simulink model "robotPrototype"  (R2021a)
settings: Solver=ode15s  StartTime=0.0  StopTime=simTime
model workspace: external: MAT-File (data not in the file)
values from neighbouring files (symbols this model uses):
  controlLim = [0.15 3 3]    [simulinkModelParam.mat]
  controlWeight = [0.75 0.6 0.5]    [simulinkModelParam.mat]
  delta = 0.3    [robotParameters.m]    (also in simulinkModelParam.mat = 0.25)
  deltaPlus = 0.20    (= 0.2)    [robotParameters.m]    (also in simulinkModelParam.mat = 0.15)
  den_CoP = [1 -1.84477840502 0.855986791935]    [simulinkModelParam.mat]
  den_zddot = [1 -1.92894226325 0.931381682127]    [simulinkModelParam.mat]
  f_0 = [1,1; deltaPlus-CoM_0(1), -(delta-deltaPlus+CoM_0(1))]\[m*9.81/2;0]    [robotParameters.m]
  f_sample = 500    [robotParameters.m]    (also in simulinkModelParam.mat = 1000)
  filterCoef = 50    [robotParameters.m]    (also in simulinkModelParam.mat = 1000)
  foot_x = delta    (= 0.3)    [robotParameters.m]    (also in simulinkModelParam.mat = 0.25)
  foot_y = delta/3    (= 0.1)    [robotParameters.m]    (also in simulinkModelParam.mat = 0.0833333333333)
  foot_z = 0.03    [robotParameters.m]    (also in simulinkModelParam.mat = 0.02)
  kd_ank = 0    [robotParameters.m]    (also in simulinkModelParam.mat)
  kd_hip = 250    [robotParameters.m]    (also in simulinkModelParam.mat = 12)
  kd_knee1 = 0.02    [robotParameters.m]    (also in simulinkModelParam.mat = 0)
  kd_knee2 = 500    [robotParameters.m]    (also in simulinkModelParam.mat = 150)
  ki_ank = 1800    [robotParameters.m]    (also in simulinkModelParam.mat = 500)
  ki_hip = 0    [robotParameters.m]    (also in simulinkModelParam.mat)
  ki_knee1 = 0    [robotParameters.m]    (also in simulinkModelParam.mat = 0.5)
  ki_knee2 = 0    [robotParameters.m]    (also in simulinkModelParam.mat)
  kp_ank = 375    [robotParameters.m]    (also in simulinkModelParam.mat = 325)
  kp_hip = 500    [robotParameters.m]    (also in simulinkModelParam.mat = 25)
  kp_knee1 = 8    [robotParameters.m]    (also in simulinkModelParam.mat = 3)
  kp_knee2 = 1000    [robotParameters.m]    (also in simulinkModelParam.mat = 300)
  L = 0.94*2*legLength    (= 0.7896)    [robotParameters.m]    (also in simulinkModelParam.mat = 0.72)
  legLength = param(1)    [forwardKin.m]    (also in robotParameters.m = 0.42; simulinkModelParam.mat = 0.4)
  legWidth = 0.08    [robotParameters.m]    (also in simulinkModelParam.mat = 0.05)
  limbThickness = 0.05    [robotParameters.m]    (also in simulinkModelParam.mat = 0.025)
  m = param(3)    [forwardKin.m]    (also in robotParameters.m = 70; simulinkModelParam.mat = 25)
  modelProperties = [25 0.5781 0.72]    [simulinkModelParam.mat]
  N = length(theta)    [robotParameters.m]
  num_CoP = [0.00280209672777 0.00560419345555 0.00280209672777]    [simulinkModelParam.mat]
  num_zddot = [0.000609854718717 0.00121970943743 0.000609854718717]    [simulinkModelParam.mat]
  p = 28    [simulinkModelParam.mat]
  pushDur = 0.1    [compareReducedOrderModels.m]    (also in simulinkModelParam.mat; startUpBalanceRobot.m)
  pushForce = pushForce - 2*pushStep    (= 0)    [compareReducedOrderModels.m]    (also in startUpBalanceRobot.m = 494)
  pushOnset = 0.2    [compareReducedOrderModels.m]    (also in simulinkModelParam.mat; startUpBalanceRobot.m)
  segmentMass = struct('torso',0.681, 'thigh', 0.2, 'shank', 0.09, 'foot', 0.029)    [robotParameters.m]
  stateLim = [0.15 1.57079632679 0.8 0.55 1.622 0.3]    [simulinkModelParam.mat]
  stateWeight = [3 0.5 0.3 9 0.25 0.09]    [simulinkModelParam.mat]
  support_x = 2.5    [robotParameters.m]    (also in simulinkModelParam.mat)
  support_y = 2.5    [robotParameters.m]    (also in simulinkModelParam.mat)
  support_z = 0.1    [robotParameters.m]    (also in simulinkModelParam.mat)
  torsoCoM = param(2)    [forwardKin.m]    (also in robotParameters.m = 0.235; simulinkModelParam.mat = 0.1875)
  torsoLength = 0.47    [robotParameters.m]    (also in simulinkModelParam.mat = 0.25)
  zmax = (2*legLength)*sin(acos(0.2/(2*legLength)))+ankleOffset    [robotParameters.m]    (also in simulinkModelParam.mat = 0.8)
  zmin = 0.6+ ankleOffset    (= 0.67)    [robotParameters.m]    (also in simulinkModelParam.mat = 0.6)
undefined symbols (not defined in the file or in its folder): controlRateWeight, den_qdot, nlobjLIP, num_qdot, X, Y, Z
libraries: sm_lib x27, nesl_utility x19, pid_lib x16, robotmaniplib x16, simulink_extras x16, mpclib x4, Contact_Forces_Lib x4, simulink x2
(part 2 of 3)

== system robotPrototype/Robot/Torso ==
  CoM to Hip : sm_lib/Frames and Transforms/Rigid Transform  TranslationMethod=StandardAxis  TranslationStandardOffset=torsoLength-torsoCoM  TranslationLengthUnit=m  TranslationStandardAxis=-Z  TranslationCartesianOffset=[0 0 0]  TranslationROffset=0  TranslationROffsetUnits=m  TranslationZOffset=0  TranslationZOffsetUnits=m  TranslationThetaOffset=0  TranslationThetaOffsetUnits=deg  RotationMethod=StandardAxis  RotationAngleUnits=deg  RotationStandardAxis=+X  RotationAngle=0  RotationArbitraryAxis=[0 0 1]  FollAlignAxisA=+X  BaseAlignAxisA=+Y  FollAlignAxisB=+Y  BaseAlignAxisB=+Z  RotationSequenceAxes=FollowerAxes  RotationSequence=XYX  RotationSequenceAngles=[0 0 0]  RotationSequenceAnglesUnits=deg  RotationMatrix=[1 0 0; 0 1 0; 0 0 1]
  CoM torso : sm_lib/Frames and Transforms/Rigid Transform  TranslationMethod=StandardAxis  TranslationStandardOffset=torsoCoM  TranslationLengthUnit=m  TranslationStandardAxis=-Y  TranslationCartesianOffset=[0 0 0]  TranslationROffset=0  TranslationROffsetUnits=m  TranslationZOffset=0  TranslationZOffsetUnits=m  TranslationThetaOffset=0  TranslationThetaOffsetUnits=deg  RotationMethod=StandardAxis  RotationAngleUnits=deg  RotationStandardAxis=+X  RotationAngle=-90  RotationArbitraryAxis=[0 0 1]  FollAlignAxisA=+X  BaseAlignAxisA=+Y  FollAlignAxisB=+Y  BaseAlignAxisB=+Z  RotationSequenceAxes=FollowerAxes  RotationSequence=XYX  RotationSequenceAngles=[0 0 0]  RotationSequenceAnglesUnits=deg  RotationMatrix=[1 0 0; 0 1 0; 0 0 1]
  Hip to joint orientation : sm_lib/Frames and Transforms/Rigid Transform  TranslationMethod=None  TranslationStandardOffset=0  TranslationLengthUnit=m  TranslationStandardAxis=+Z  TranslationCartesianOffset=[0 0 0]  TranslationROffset=0  TranslationROffsetUnits=m  TranslationZOffset=0  TranslationZOffsetUnits=m  TranslationThetaOffset=0  TranslationThetaOffsetUnits=deg  RotationMethod=StandardAxis  RotationAngleUnits=deg  RotationStandardAxis=+X  RotationAngle=90  RotationArbitraryAxis=[0 0 1]  FollAlignAxisA=+X  BaseAlignAxisA=+Y  FollAlignAxisB=+Y  BaseAlignAxisB=+Z  RotationSequenceAxes=FollowerAxes  RotationSequence=XYX  RotationSequenceAngles=[0 0 0]  RotationSequenceAnglesUnits=deg  RotationMatrix=[1 0 0; 0 1 0; 0 0 1]
  Planar Joint to Torso : sm_lib/Frames and Transforms/Rigid Transform  TranslationMethod=None  TranslationStandardOffset=0  TranslationLengthUnit=m  TranslationStandardAxis=+Z  TranslationCartesianOffset=[0 0 0]  TranslationROffset=0  TranslationROffsetUnits=m  TranslationZOffset=0  TranslationZOffsetUnits=m  TranslationThetaOffset=0  TranslationThetaOffsetUnits=deg  RotationMethod=None  RotationAngleUnits=deg  RotationStandardAxis=+Z  RotationAngle=0.0  RotationArbitraryAxis=[0 0 1]  FollAlignAxisA=+X  BaseAlignAxisA=+Y  FollAlignAxisB=+Y  BaseAlignAxisB=+Z  RotationSequenceAxes=FollowerAxes  RotationSequence=XYX  RotationSequenceAngles=[0 0 0]  RotationSequenceAnglesUnits=deg  RotationMatrix=[1 0 0; 0 1 0; 0 0 1]
  Torso : sm_lib/Body Elements/Extruded Solid  GraphicAmbientColor=[0.15 0.15 0.15 1.0]  BasedOnType=Mass  CenterOfMass=[0 -torsoCoM 0]  CenterOfMassUnits=m  GraphicDiffuseColor=[0.0 0.0 1.0]  ExportConvexHullGeometry=off  ExtrusionCrossSection=torso_xy  ExtrusionCrossSectionUnits=m  Density=1000  DensityUnits=kg/m^3  DoExposeReferenceFrame=on  GraphicEmissiveColor=[0.0 0.0 0.0 1.0]  ExportEntireGeometry=off  ExtrusionLength=limbThickness+0.02  ExtrusionLengthUnits=m  ExtrusionType=General  SerializedFrames=<Frames/>  MarkerShape=Sphere  MarkerSize=10  GraphicType=FromGeometry  InertiaType=Custom  Mass=segmentMass.torso*m  MassUnits=kg  MomentsOfInertia=[1.367 0.094 (8 - segmentMass.torso*m*(torsoCoM)^2 )]  MomentsOfInertiaUnits=kg*m^2  PolygonNumSides=3  GraphicOpacity=1.0  PolygonOuterRadius=1  PolygonOuterRadiusUnits=m  ProductsOfInertia=[0 0 0]  ProductsOfInertiaUnits=kg*m^2  GraphicShininess=75  GraphicSpecularColor=[0.5 0.5 0.5 1.0]  GraphicVisPropType=SimpleVisualProperties
  Hip Frame : PMIOPort  Side=Left
  Planar Joint : PMIOPort  Port=2  Side=Left
  Hip Joint : PMIOPort  Port=3  Side=Right
  Disturbance : PMIOPort  Port=4  Side=Left
  connections:
  Torso/RConn1 -- Planar Joint to Torso/RConn1 -- CoM torso/LConn1
  Hip Frame/RConn1 -- Disturbance/RConn1 -- Hip to joint orientation/LConn1 -- CoM to Hip/RConn1
  Planar Joint to Torso/LConn1 -- Planar Joint/RConn1
  CoM to Hip/LConn1 -- CoM torso/RConn1
  Hip Joint/RConn1 -- Hip to joint orientation/RConn1

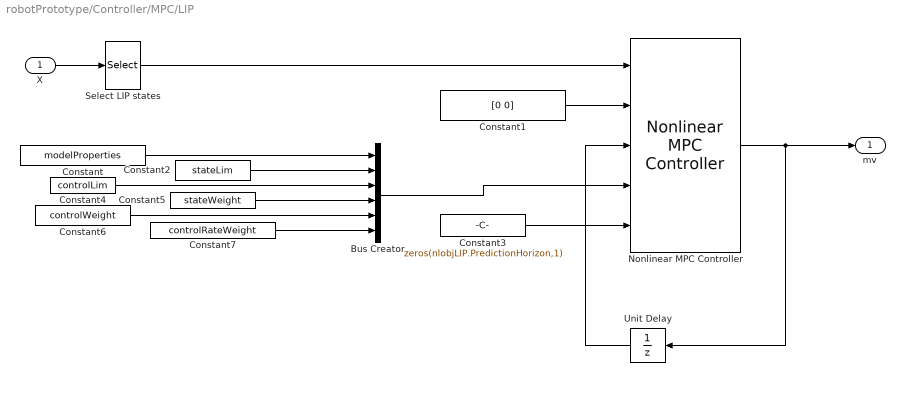
== system robotPrototype/Controller/MPC/LIP ==
  X : Inport
  Bus Creator : BusCreator  Inputs=6  OutDataTypeStr=Bus: myBusObjectLIP  NonVirtualBus=on
      settings: InheritFromInputs=off
  Constant : Constant  Value=modelProperties
  Constant1 : Constant  Value=[0 0]  VectorParams1D=off  OutDataTypeStr=double
  Constant2 : Constant  Value=stateLim
  Constant3 : Constant  Value=zeros(nlobjLIP.PredictionHorizon,1)
  Constant4 : Constant  Value=controlLim
  Constant5 : Constant  Value=stateWeight
  Constant6 : Constant  Value=controlWeight
  Constant7 : Constant  Value=controlRateWeight
  Nonlinear MPC Controller : mpclib/Nonlinear MPC Controller  SCDEnableBlockLinearizationSpecification=on  nlmpcobj=nlobjLIP  UseObjectTs=on  UseMEX=off  md_enabled=off  mvtarget_enabled=on  param_enabled=on  cost_enabled=off  mvseq_enabled=off  stateseq_enabled=off  ovseq_enabled=off  slack_enabled=off  status_enabled=off  ov_min=off  ov_max=off  mv_min=off  mv_max=off  mvrate_min=off  mvrate_max=off  state_min=off  state_max=off  ov_weight=off  mv_weight=off  mvrate_weight=off  ecr_weight=off  nlp_initialize=off
  Select LIP states : Selector  InputPortWidth=6  IndexOptions=Index vector (dialog)  Indices=[1 4]  OutputSizes=1
  Unit Delay : UnitDelay  SampleTime=-1  HasFrameUpgradeWarning=on
  mv : Outport
  wires:
  Bus Creator/1 -> Nonlinear MPC Controller/4
  Constant3/1 -> Nonlinear MPC Controller/5
  Unit Delay/1 -> Nonlinear MPC Controller/3
  Constant1/1 -> Nonlinear MPC Controller/2
  Nonlinear MPC Controller/1 -> Unit Delay/1, mv/1
  X/1 -> Select LIP states/1
  Select LIP states/1 -> Nonlinear MPC Controller/1
  Constant5/1 -> Bus Creator/4
  Constant4/1 -> Bus Creator/3
  Constant2/1 -> Bus Creator/2
  Constant/1 -> Bus Creator/1
  Constant6/1 -> Bus Creator/5
  Constant7/1 -> Bus Creator/6

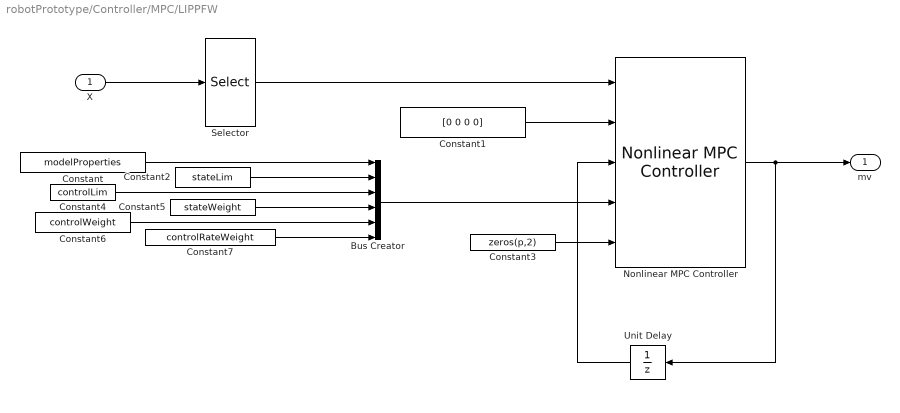
== system robotPrototype/Controller/MPC/LIPPFW ==
  X : Inport
  Bus Creator : BusCreator  Inputs=6  OutDataTypeStr=Bus: myBusObjectLIPPFW  NonVirtualBus=on
      settings: InheritFromInputs=off
  Constant : Constant  Value=modelProperties
  Constant1 : Constant  Value=[0 0 0 0]  VectorParams1D=off  OutDataTypeStr=double
  Constant2 : Constant  Value=stateLim
  Constant3 : Constant  Value=zeros(p,2)
  Constant4 : Constant  Value=controlLim
  Constant5 : Constant  Value=stateWeight
  Constant6 : Constant  Value=controlWeight
  Constant7 : Constant  Value=controlRateWeight
  Nonlinear MPC Controller : mpclib/Nonlinear MPC Controller  SCDEnableBlockLinearizationSpecification=on  nlmpcobj=nlobjLIPPFW  UseObjectTs=on  UseMEX=off  md_enabled=off  mvtarget_enabled=on  param_enabled=on  cost_enabled=off  mvseq_enabled=off  stateseq_enabled=off  ovseq_enabled=off  slack_enabled=off  status_enabled=off  ov_min=off  ov_max=off  mv_min=off  mv_max=off  mvrate_min=off  mvrate_max=off  state_min=off  state_max=off  ov_weight=off  mv_weight=off  mvrate_weight=off  ecr_weight=off  nlp_initialize=off
  Selector : Selector  InputPortWidth=6  IndexOptions=Index vector (dialog)  Indices=[1 2 4 5]  OutputSizes=1
  Unit Delay : UnitDelay  SampleTime=-1  HasFrameUpgradeWarning=on
  mv : Outport
  wires:
  Unit Delay/1 -> Nonlinear MPC Controller/3
  Constant1/1 -> Nonlinear MPC Controller/2
  Nonlinear MPC Controller/1 -> mv/1, Unit Delay/1
  Bus Creator/1 -> Nonlinear MPC Controller/4
  Constant3/1 -> Nonlinear MPC Controller/5
  Constant5/1 -> Bus Creator/4
  Constant4/1 -> Bus Creator/3
  Constant2/1 -> Bus Creator/2
  Constant/1 -> Bus Creator/1
  Constant6/1 -> Bus Creator/5
  X/1 -> Selector/1
  Selector/1 -> Nonlinear MPC Controller/1
  Constant7/1 -> Bus Creator/6

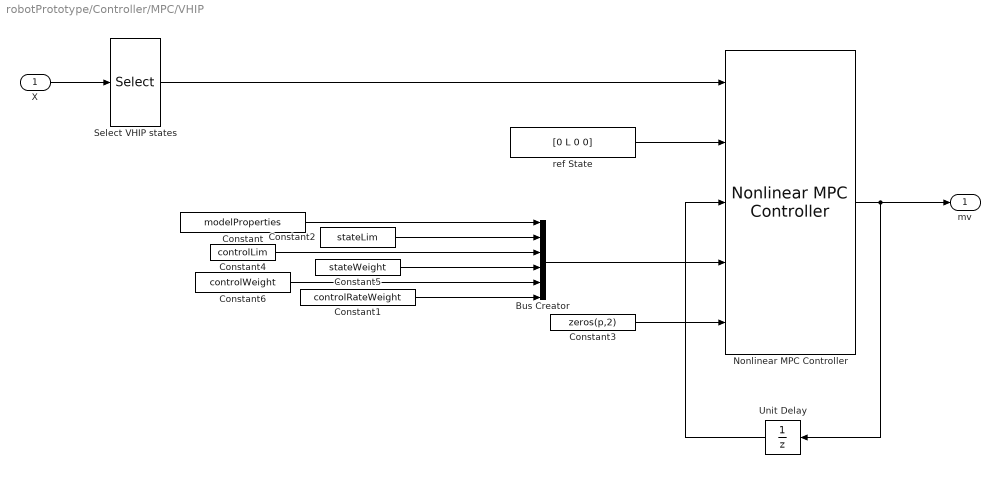
== system robotPrototype/Controller/MPC/VHIP ==
  X : Inport
  Bus Creator : BusCreator  Inputs=6  OutDataTypeStr=Bus: myBusObjectVHIP  NonVirtualBus=on
      settings: InheritFromInputs=off
  Constant : Constant  Value=modelProperties
  Constant1 : Constant  Value=controlRateWeight
  Constant2 : Constant  Value=stateLim
  Constant3 : Constant  Value=zeros(p,2)
  Constant4 : Constant  Value=controlLim
  Constant5 : Constant  Value=stateWeight
  Constant6 : Constant  Value=controlWeight
  Nonlinear MPC Controller : mpclib/Nonlinear MPC Controller  SCDEnableBlockLinearizationSpecification=on  nlmpcobj=nlobjVHIP  UseObjectTs=on  UseMEX=off  md_enabled=off  mvtarget_enabled=on  param_enabled=on  cost_enabled=off  mvseq_enabled=off  stateseq_enabled=off  ovseq_enabled=off  slack_enabled=off  status_enabled=off  ov_min=off  ov_max=off  mv_min=off  mv_max=off  mvrate_min=off  mvrate_max=off  state_min=off  state_max=off  ov_weight=off  mv_weight=off  mvrate_weight=off  ecr_weight=off  nlp_initialize=off
  Select VHIP states : Selector  InputPortWidth=6  IndexOptions=Index vector (dialog)  Indices=[1 3 4 6]  OutputSizes=1
  Unit Delay : UnitDelay  SampleTime=-1  HasFrameUpgradeWarning=on
  ref State : Constant  Value=[0 L 0 0]  VectorParams1D=off  OutDataTypeStr=double
  mv : Outport
  wires:
  Unit Delay/1 -> Nonlinear MPC Controller/3
  ref State/1 -> Nonlinear MPC Controller/2
  Nonlinear MPC Controller/1 -> Unit Delay/1, mv/1
  Bus Creator/1 -> Nonlinear MPC Controller/4
  Constant3/1 -> Nonlinear MPC Controller/5
  X/1 -> Select VHIP states/1
  Select VHIP states/1 -> Nonlinear MPC Controller/1
  Constant5/1 -> Bus Creator/4
  Constant/1 -> Bus Creator/1
  Constant4/1 -> Bus Creator/3
  Constant2/1 -> Bus Creator/2
  Constant6/1 -> Bus Creator/5
  Constant1/1 -> Bus Creator/6

== system robotPrototype/Controller/MPC/VHIPPFW ==
  X : Inport
  Bus Creator : BusCreator  Inputs=6  OutDataTypeStr=Bus: myBusObjectVHIPPFW  NonVirtualBus=on
      settings: InheritFromInputs=off
  Constant : Constant  Value=modelProperties
  Constant1 : Constant  Value=controlRateWeight
  Constant2 : Constant  Value=stateLim
  Constant3 : Constant  Value=zeros(p,3)
  Constant4 : Constant  Value=controlLim
  Constant5 : Constant  Value=stateWeight
  Constant6 : Constant  Value=controlWeight
  Nonlinear MPC Controller : mpclib/Nonlinear MPC Controller  SCDEnableBlockLinearizationSpecification=on  nlmpcobj=nlobjVHIPPFW  UseObjectTs=on  UseMEX=off  md_enabled=off  mvtarget_enabled=on  param_enabled=on  cost_enabled=off  mvseq_enabled=off  stateseq_enabled=off  ovseq_enabled=off  slack_enabled=off  status_enabled=off  ov_min=off  ov_max=off  mv_min=off  mv_max=off  mvrate_min=off  mvrate_max=off  state_min=off  state_max=off  ov_weight=off  mv_weight=off  mvrate_weight=off  ecr_weight=off  nlp_initialize=off
  Unit Delay : UnitDelay  SampleTime=-1  HasFrameUpgradeWarning=on
  refState : Constant  Value=[0 0 L 0 0 0]  VectorParams1D=off  OutDataTypeStr=double
  mv : Outport
  wires:
  Bus Creator/1 -> Nonlinear MPC Controller/4
  Constant3/1 -> Nonlinear MPC Controller/5
  Constant2/1 -> Bus Creator/2
  Constant/1 -> Bus Creator/1
  X/1 -> Nonlinear MPC Controller/1
  Unit Delay/1 -> Nonlinear MPC Controller/3
  refState/1 -> Nonlinear MPC Controller/2
  Nonlinear MPC Controller/1 -> mv/1, Unit Delay/1
  Constant4/1 -> Bus Creator/3
  Constant5/1 -> Bus Creator/4
  Constant6/1 -> Bus Creator/5
  Constant1/1 -> Bus Creator/6

== system robotPrototype/Controller/Variant Subsystem/LIP ==
  mv : Inport
  measureData : Inport  Port=2
  Bus Creator : BusCreator  Inputs=3
  Bus Selector : BusSelector  OutputSignals=CoP,jointPos,state,ContactForces,jointAng
  Demux2 : Demux  Outputs=3
  Feedback Correction : Subsystem
  Inverse Dynamics1 : Subsystem
  jointTorque : Outport
  wires:
  measureData/1 -> Bus Selector/1
  Demux2/1 -> Bus Creator/1  "ankle"
  Demux2/2 -> Bus Creator/2  "knee"
  Demux2/3 -> Bus Creator/3  "hip"
  Bus Creator/1 -> jointTorque/1
  mv/1 -> Feedback Correction/1(mpc controls)
  Bus Selector/1 -> Feedback Correction/2(<CoP>)  "<CoP>"
  Bus Selector/2 -> Feedback Correction/3(<jointPos>)  "<jointPos>"
  Bus Selector/3 -> Feedback Correction/4(<state>)  "<state>"
  Feedback Correction/1(tau correction) -> Inverse Dynamics1/1(tau corrective)
  Inverse Dynamics1/1(tau compesation) -> Demux2/1
  Bus Selector/5 -> Inverse Dynamics1/2(<jointAng>)  "<jointAng>"
  Bus Selector/4 -> Feedback Correction/5(footContact)  "<ContactForces>"

== system robotPrototype/Controller/Variant Subsystem/LIPPFW ==
  mv : Inport
  measureData : Inport  Port=2
  Bus Creator : BusCreator  Inputs=3
  Bus Selector : BusSelector  OutputSignals=CoP,jointPos,jointAng,ContactForces
  Demux : Demux  Outputs=3
  Feedback Compensation : Subsystem
  Inverse Dynamics : Subsystem
  jointTorque : Outport
  wires:
  measureData/1 -> Bus Selector/1
  Bus Creator/1 -> jointTorque/1
  Demux/3 -> Bus Creator/3  "hip"
  mv/1 -> Feedback Compensation/1(mpc control)
  Bus Selector/1 -> Feedback Compensation/2(<CoP>)  "<CoP>"
  Bus Selector/2 -> Feedback Compensation/3(<jointPos>)  "<jointPos>"
  Demux/1 -> Bus Creator/1  "ankle"
  Demux/2 -> Bus Creator/2  "knee"
  Feedback Compensation/1(tau corrective) -> Inverse Dynamics/1(tau corrective)
  Inverse Dynamics/1(tau compesation) -> Demux/1
  Bus Selector/3 -> Inverse Dynamics/2(<jointAng>)  "<jointAng>"
  Bus Selector/4 -> Feedback Compensation/4(Heal Normal Force)  "<ContactForces>"

== system robotPrototype/Controller/Variant Subsystem/VHIP ==
  mv : Inport
  measureData : Inport  Port=2
  Bus Creator : BusCreator  Inputs=3
  Bus Selector : BusSelector  OutputSignals=state,CoP,zddot,ContactForces,jointAng
  Demux2 : Demux  Outputs=3
  Feedback Correction : Subsystem
  Inverse Dynamics : Subsystem
  jointTorque : Outport
  wires:
  measureData/1 -> Bus Selector/1
  Bus Creator/1 -> jointTorque/1
  Demux2/1 -> Bus Creator/1  "ankle"
  Demux2/2 -> Bus Creator/2  "knee"
  Demux2/3 -> Bus Creator/3  "hip"
  mv/1 -> Feedback Correction/1(mpc controls)
  Bus Selector/1 -> Feedback Correction/2(<state>)  "<state>"
  Bus Selector/2 -> Feedback Correction/3(<CoP>)  "<CoP>"
  Bus Selector/3 -> Feedback Correction/4(<zddot>)  "<zddot>"
  Bus Selector/5 -> Inverse Dynamics/2(<jointAng>)  "<jointAng>"
  Inverse Dynamics/1(tau compesation) -> Demux2/1
  Feedback Correction/1(Tau correction) -> Inverse Dynamics/1(tau corrective)
  Bus Selector/4 -> Feedback Correction/5(footContact)  "<ContactForces>"

== system robotPrototype/Controller/Variant Subsystem/VIPPFW ==
  mv : Inport
  measureData : Inport  Port=2
  Bus Creator : BusCreator  Inputs=3
  Bus Selector : BusSelector  OutputSignals=CoP,zddot,jointPos,ContactForces,jointAng
  Bus Selector1 : BusSelector  OutputSignals=X_hip
  Demux : Demux  Outputs=3
  Demux1 : Demux  Outputs=2
  Inverse Dynamics : Subsystem
  Terminator : Terminator
  feedback correction : Subsystem
  jointTorque : Outport
  wires:
  Bus Creator/1 -> jointTorque/1
  measureData/1 -> Bus Selector/1
  Bus Selector/5 -> Inverse Dynamics/2(<jointAng>)  "<jointAng>"
  mv/1 -> feedback correction/1(mpc controls)
  Bus Selector/1 -> feedback correction/2(<CoP>)  "<CoP>"
  Bus Selector/2 -> feedback correction/3(<zddot>)  "<zddot>"
  Demux/1 -> Bus Creator/1  "ankle"
  Demux/2 -> Bus Creator/2  "knee"
  Demux/3 -> Bus Creator/3  "hip"
  Bus Selector/3 -> Bus Selector1/1  "<jointPos>"
  Bus Selector1/1 -> Demux1/1  "<X_hip>"
  Demux1/1 -> Terminator/1
  Demux1/2 -> feedback correction/4(z)
  Inverse Dynamics/1(tau compesation) -> Demux/1
  feedback correction/1(tau correction) -> Inverse Dynamics/1(tau corrective)
  Bus Selector/4 -> feedback correction/5(footContact)  "<ContactForces>"

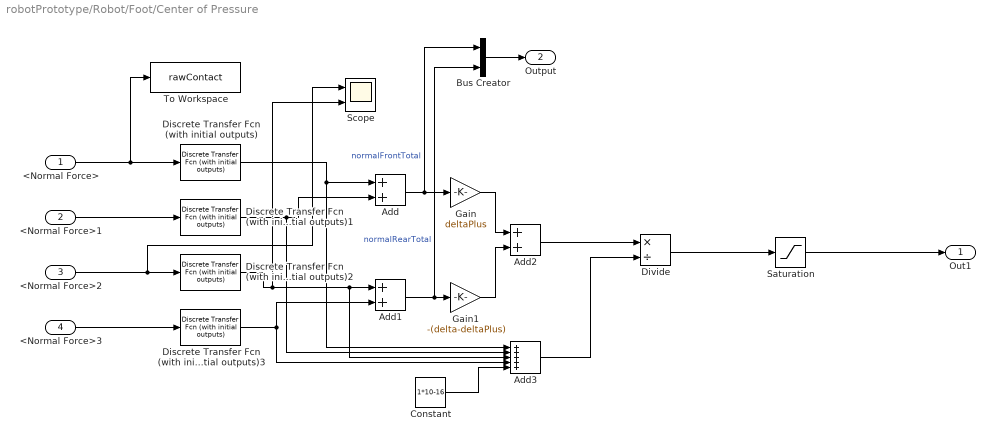
== system robotPrototype/Robot/Foot/Center of Pressure ==
  <Normal Force> : Inport
  <Normal Force>1 : Inport  Port=2
  <Normal Force>2 : Inport  Port=3
  <Normal Force>3 : Inport  Port=4
  Add : Sum
  Add1 : Sum
  Add2 : Sum
  Add3 : Sum  Inputs=+++++
  Bus Creator : BusCreator  Inputs=2
  Constant : Constant  Value=1*10-16
  Discrete Transfer Fcn (with initial outputs) : simulink_extras/Additional Discrete/Discrete Transfer Fcn (with initial outputs)  N=num_CoP  D=den_CoP  U0=0  Y0=f_0(1)  TS=1/f_sample
      settings: SourceProductBaseCode=SL
  Discrete Transfer Fcn (with initial outputs)1 : simulink_extras/Additional Discrete/Discrete Transfer Fcn (with initial outputs)  N=num_CoP  D=den_CoP  U0=0  Y0=f_0(1)  TS=1/f_sample
      settings: SourceProductBaseCode=SL
  Discrete Transfer Fcn (with initial outputs)2 : simulink_extras/Additional Discrete/Discrete Transfer Fcn (with initial outputs)  N=num_CoP  D=den_CoP  U0=0  Y0=f_0(2)  TS=1/f_sample
      settings: SourceProductBaseCode=SL
  Discrete Transfer Fcn (with initial outputs)3 : simulink_extras/Additional Discrete/Discrete Transfer Fcn (with initial outputs)  N=num_CoP  D=den_CoP  U0=0  Y0=f_0(2)  TS=1/f_sample
      settings: SourceProductBaseCode=SL
  Divide : Product  Inputs=*/
  Gain : Gain  Gain=deltaPlus
  Gain1 : Gain  Gain=-(delta-deltaPlus)
  Saturation : Saturate  UpperLimit=deltaPlus  LowerLimit=-(delta-deltaPlus)
  Scope : Scope  NumInputPorts=2
  To Workspace : ToWorkspace  VariableName=rawContact  SaveFormat=Timeseries  SampleTime=1/f_sample
  Out1 : Outport
  Output : Outport  Port=2
  wires:
  Gain/1 -> Add2/1
  Add1/1 -> Bus Creator/2, Gain1/1  "normalRearTotal"
  <Normal Force>3/1 -> Discrete Transfer Fcn (with initial outputs)3/1
  <Normal Force>1/1 -> Discrete Transfer Fcn (with initial outputs)1/1
  <Normal Force>2/1 -> Scope/1, Discrete Transfer Fcn (with initial outputs)2/1
  Add3/1 -> Divide/2
  Add/1 -> Bus Creator/1, Gain/1  "normalFrontTotal"
  <Normal Force>/1 -> Discrete Transfer Fcn (with initial outputs)/1, To Workspace/1
  Gain1/1 -> Add2/2
  Add2/1 -> Divide/1
  Discrete Transfer Fcn (with initial outputs)2/1 -> Scope/2, Add3/3, Add1/1
  Discrete Transfer Fcn (with initial outputs)3/1 -> Add1/2, Add3/4
  Discrete Transfer Fcn (with initial outputs)1/1 -> Add/2, Add3/2
  Discrete Transfer Fcn (with initial outputs)/1 -> Add3/1, Add/1
  Bus Creator/1 -> Output/1
  Constant/1 -> Add3/5
  Divide/1 -> Saturation/1
  Saturation/1 -> Out1/1

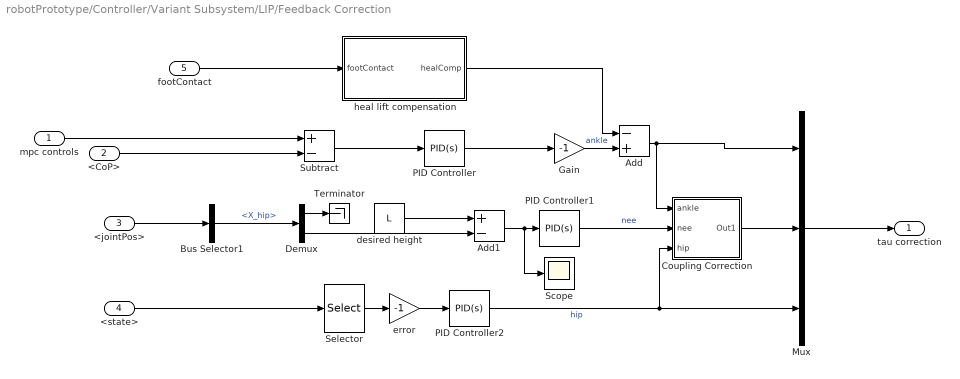
== system robotPrototype/Controller/Variant Subsystem/LIP/Feedback Correction ==
  mpc controls : Inport
  <CoP> : Inport  Port=2
  <jointPos> : Inport  Port=3
  <state> : Inport  Port=4
  footContact : Inport  Port=5
  Add : Sum  Inputs=-+
  Add1 : Sum  Inputs=+-
  Bus Selector1 : BusSelector  OutputSignals=X_hip
  Coupling Correction : Subsystem
  Demux : Demux  Outputs=2
  Gain : Gain  Gain=-1
  Mux : Mux  Inputs=3
  PID Controller : pid_lib/PID Controller  Controller=PID  Form=Parallel  TimeDomain=Continuous-time  UseExternalTs=off  SampleTime=-1  IntegratorMethod=Forward Euler  FilterMethod=Forward Euler  ControllerParametersSource=internal  P=kp_ank  I=ki_ank  D=kd_ank  UseFilter=on  N=filterCoef  TunerSelectOption=Transfer Function Based (PID Tuner App)  InitialConditionSource=internal  InitialConditionForIntegrator=0  InitialConditionForFilter=0  DifferentiatorICPrevScaledInput=0  ExternalReset=none  TrackingMode=off  Kt=1  LimitOutput=off  SatLimitsSource=internal  UpperSaturationLimit=inf  LowerSaturationLimit=-inf  LinearizeAsGain=on  AntiWindupMode=none  Kb=1  POutMin=[]  POutMax=[]  IOutMin=[]  IOutMax=[]  DOutMin=[]  DOutMax=[]  NOutMin=[]  NOutMax=[]  SumOutMin=[]  SumOutMax=[]  SaturationOutMin=[]  SaturationOutMax=[]  PParamMin=[]  PParamMax=[]  IParamMin=[]  IParamMax=[]  DParamMin=[]  DParamMax=[]  NParamMin=[]  NParamMax=[]  KbParamMin=[]  KbParamMax=[]  KtParamMin=[]  KtParamMax=[]  KbOutMin=[]  KbOutMax=[]  KtOutMin=[]  KtOutMax=[]  IntegratorOutMin=[]  IntegratorOutMax=[]  FilterOutMin=[]  FilterOutMax=[]  SumI1OutMin=[]  SumI1OutMax=[]  SumI2OutMin=[]  SumI2OutMax=[]  SumI3OutMin=[]  SumI3OutMax=[]  SumI4OutMin=[]  SumI4OutMax=[]  SumDOutMin=[]  SumDOutMax=[]  DifferentiatorOutMin=[]  DifferentiatorOutMax=[]  FilterDiffOutCoefMin=[]  FilterDiffOutCoefMax=[]  ReciprocalOutMin=[]  ReciprocalOutMax=[]  SumDenOutMin=[]  SumDenOutMax=[]  SumNumOutMin=[]  SumNumOutMax=[]  DivideOutMin=[]  DivideOutMax=[]  UdiffTsProdOutMin=[]  UdiffTsProdOutMax=[]  NTsProdOutMin=[]  NTsProdOutMax=[]  UintegralTsProdOutMin=[]  UintegralTsProdOutMax=[]  UngainTsProdOutMin=[]  UngainTsProdOutMax=[]  IntegratorContinuousStateAttributes=''  IntegratorStateMustResolveToSignalObject=off  IntegratorRTWStateStorageClass=Auto  FilterContinuousStateAttributes=''  FilterStateMustResolveToSignalObject=off  FilterRTWStateStorageClass=Auto  ParallelPVariant=InternalParameters  IdealPVariant=Disabled  IVariant=InternalParameters  DVariant=InternalParameters  IntegratorVariant=Continuous  SatVariant=Disabled  AWVariant=Passthrough  PCopyVariant=Disabled  TRVariant=Disabled  FdbkBlocksVariant=Forward  IdealPFdbkVariant=Disabled  SatFdbkVariant=Disabled  DerivativeFilterVariant=ContFilter  NVariant=InternalParameters  NCopyVariant=Disabled  FilterICVariant=InternalICsFilter  IntegratorICVariant=InternalICs  ExternalResetVariant=Disabled  TRSumVariant=Passthrough  SumFdbkVariant=Disabled  SumVariant=Sum_PID  TsampFilterVariant=InternalTs  TsampNgainVariant=Passthrough  TsampIntegralVariant=Passthrough  ExternalSaturationOutDataTypeStr=Inherit: Same as second input
  PID Controller1 : pid_lib/PID Controller  Controller=PID  Form=Parallel  TimeDomain=Continuous-time  UseExternalTs=off  SampleTime=-1  IntegratorMethod=Forward Euler  FilterMethod=Forward Euler  ControllerParametersSource=internal  P=kp_knee2  I=ki_knee2  D=kd_knee2  UseFilter=on  N=filterCoef  TunerSelectOption=Transfer Function Based (PID Tuner App)  InitialConditionSource=internal  InitialConditionForIntegrator=0  InitialConditionForFilter=0  DifferentiatorICPrevScaledInput=0  ExternalReset=none  TrackingMode=off  Kt=1  LimitOutput=off  SatLimitsSource=internal  UpperSaturationLimit=inf  LowerSaturationLimit=-inf  LinearizeAsGain=on  AntiWindupMode=none  Kb=1  POutMin=[]  POutMax=[]  IOutMin=[]  IOutMax=[]  DOutMin=[]  DOutMax=[]  NOutMin=[]  NOutMax=[]  SumOutMin=[]  SumOutMax=[]  SaturationOutMin=[]  SaturationOutMax=[]  PParamMin=[]  PParamMax=[]  IParamMin=[]  IParamMax=[]  DParamMin=[]  DParamMax=[]  NParamMin=[]  NParamMax=[]  KbParamMin=[]  KbParamMax=[]  KtParamMin=[]  KtParamMax=[]  KbOutMin=[]  KbOutMax=[]  KtOutMin=[]  KtOutMax=[]  IntegratorOutMin=[]  IntegratorOutMax=[]  FilterOutMin=[]  FilterOutMax=[]  SumI1OutMin=[]  SumI1OutMax=[]  SumI2OutMin=[]  SumI2OutMax=[]  SumI3OutMin=[]  SumI3OutMax=[]  SumI4OutMin=[]  SumI4OutMax=[]  SumDOutMin=[]  SumDOutMax=[]  DifferentiatorOutMin=[]  DifferentiatorOutMax=[]  FilterDiffOutCoefMin=[]  FilterDiffOutCoefMax=[]  ReciprocalOutMin=[]  ReciprocalOutMax=[]  SumDenOutMin=[]  SumDenOutMax=[]  SumNumOutMin=[]  SumNumOutMax=[]  DivideOutMin=[]  DivideOutMax=[]  UdiffTsProdOutMin=[]  UdiffTsProdOutMax=[]  NTsProdOutMin=[]  NTsProdOutMax=[]  UintegralTsProdOutMin=[]  UintegralTsProdOutMax=[]  UngainTsProdOutMin=[]  UngainTsProdOutMax=[]  IntegratorContinuousStateAttributes=''  IntegratorStateMustResolveToSignalObject=off  IntegratorRTWStateStorageClass=Auto  FilterContinuousStateAttributes=''  FilterStateMustResolveToSignalObject=off  FilterRTWStateStorageClass=Auto  ParallelPVariant=InternalParameters  IdealPVariant=Disabled  IVariant=InternalParameters  DVariant=InternalParameters  IntegratorVariant=Continuous  SatVariant=Disabled  AWVariant=Passthrough  PCopyVariant=Disabled  TRVariant=Disabled  FdbkBlocksVariant=Forward  IdealPFdbkVariant=Disabled  SatFdbkVariant=Disabled  DerivativeFilterVariant=ContFilter  NVariant=InternalParameters  NCopyVariant=Disabled  FilterICVariant=InternalICsFilter  IntegratorICVariant=InternalICs  ExternalResetVariant=Disabled  TRSumVariant=Passthrough  SumFdbkVariant=Disabled  SumVariant=Sum_PID  TsampFilterVariant=InternalTs  TsampNgainVariant=Passthrough  TsampIntegralVariant=Passthrough  ExternalSaturationOutDataTypeStr=Inherit: Same as second input
  PID Controller2 : pid_lib/PID Controller  Controller=PID  Form=Parallel  TimeDomain=Continuous-time  UseExternalTs=off  SampleTime=-1  IntegratorMethod=Forward Euler  FilterMethod=Forward Euler  ControllerParametersSource=internal  P=kp_hip  I=ki_hip  D=kd_hip  UseFilter=on  N=filterCoef  TunerSelectOption=Transfer Function Based (PID Tuner App)  InitialConditionSource=internal  InitialConditionForIntegrator=0  InitialConditionForFilter=0  DifferentiatorICPrevScaledInput=0  ExternalReset=none  TrackingMode=off  Kt=1  LimitOutput=off  SatLimitsSource=internal  UpperSaturationLimit=inf  LowerSaturationLimit=-inf  LinearizeAsGain=on  AntiWindupMode=none  Kb=1  POutMin=[]  POutMax=[]  IOutMin=[]  IOutMax=[]  DOutMin=[]  DOutMax=[]  NOutMin=[]  NOutMax=[]  SumOutMin=[]  SumOutMax=[]  SaturationOutMin=[]  SaturationOutMax=[]  PParamMin=[]  PParamMax=[]  IParamMin=[]  IParamMax=[]  DParamMin=[]  DParamMax=[]  NParamMin=[]  NParamMax=[]  KbParamMin=[]  KbParamMax=[]  KtParamMin=[]  KtParamMax=[]  KbOutMin=[]  KbOutMax=[]  KtOutMin=[]  KtOutMax=[]  IntegratorOutMin=[]  IntegratorOutMax=[]  FilterOutMin=[]  FilterOutMax=[]  SumI1OutMin=[]  SumI1OutMax=[]  SumI2OutMin=[]  SumI2OutMax=[]  SumI3OutMin=[]  SumI3OutMax=[]  SumI4OutMin=[]  SumI4OutMax=[]  SumDOutMin=[]  SumDOutMax=[]  DifferentiatorOutMin=[]  DifferentiatorOutMax=[]  FilterDiffOutCoefMin=[]  FilterDiffOutCoefMax=[]  ReciprocalOutMin=[]  ReciprocalOutMax=[]  SumDenOutMin=[]  SumDenOutMax=[]  SumNumOutMin=[]  SumNumOutMax=[]  DivideOutMin=[]  DivideOutMax=[]  UdiffTsProdOutMin=[]  UdiffTsProdOutMax=[]  NTsProdOutMin=[]  NTsProdOutMax=[]  UintegralTsProdOutMin=[]  UintegralTsProdOutMax=[]  UngainTsProdOutMin=[]  UngainTsProdOutMax=[]  IntegratorContinuousStateAttributes=''  IntegratorStateMustResolveToSignalObject=off  IntegratorRTWStateStorageClass=Auto  FilterContinuousStateAttributes=''  FilterStateMustResolveToSignalObject=off  FilterRTWStateStorageClass=Auto  ParallelPVariant=InternalParameters  IdealPVariant=Disabled  IVariant=InternalParameters  DVariant=InternalParameters  IntegratorVariant=Continuous  SatVariant=Disabled  AWVariant=Passthrough  PCopyVariant=Disabled  TRVariant=Disabled  FdbkBlocksVariant=Forward  IdealPFdbkVariant=Disabled  SatFdbkVariant=Disabled  DerivativeFilterVariant=ContFilter  NVariant=InternalParameters  NCopyVariant=Disabled  FilterICVariant=InternalICsFilter  IntegratorICVariant=InternalICs  ExternalResetVariant=Disabled  TRSumVariant=Passthrough  SumFdbkVariant=Disabled  SumVariant=Sum_PID  TsampFilterVariant=InternalTs  TsampNgainVariant=Passthrough  TsampIntegralVariant=Passthrough  ExternalSaturationOutDataTypeStr=Inherit: Same as second input
  Scope : Scope
  Selector : Selector  InputPortWidth=6  IndexOptions=Index vector (dialog)  Indices=[2]  OutputSizes=1
  Subtract : Sum  Inputs=+-
  Terminator : Terminator
  desired height : Constant  Value=L
  error : Gain  Gain=-1
  heal lift compensation : Subsystem
  tau correction : Outport
  wires:
  PID Controller2/1 -> Coupling Correction/3(hip), Mux/3  "hip"
  Demux/2 -> Add1/2
  Subtract/1 -> PID Controller/1
  mpc controls/1 -> Subtract/1
  error/1 -> PID Controller2/1
  PID Controller/1 -> Gain/1
  desired height/1 -> Add1/1
  Add1/1 -> Scope/1, PID Controller1/1
  Bus Selector1/1 -> Demux/1  "<X_hip>"
  <CoP>/1 -> Subtract/2
  Selector/1 -> error/1
  Demux/1 -> Terminator/1
  <jointPos>/1 -> Bus Selector1/1
  <state>/1 -> Selector/1
  Mux/1 -> tau correction/1
  PID Controller1/1 -> Coupling Correction/2(nee)  "nee"
  Coupling Correction/1(Out1) -> Mux/2
  Gain/1 -> Add/2  "ankle"
  Add/1 -> Mux/1, Coupling Correction/1(ankle)
  heal lift compensation/1(healComp) -> Add/1
  footContact/1 -> heal lift compensation/1(footContact)

== system robotPrototype/Controller/Variant Subsystem/LIP/Inverse Dynamics1 ==
  tau corrective : Inport
  <jointAng> : Inport  Port=2
  Add : Sum  Inputs=+++
  Constant : Constant  Value=zeros(6,4)
  Forward Dynamics : robotmaniplib/Forward Dynamics  RigidBodyTree=robot  SimulateUsing=Code generation
  Gravity Torque : robotmaniplib/Gravity Torque  RigidBodyTree=robot  SimulateUsing=Code generation
  Inverse Dynamics : robotmaniplib/Inverse Dynamics  RigidBodyTree=robot  SimulateUsing=Code generation
      settings: SourceProductBaseCode=RO
  Velocity Product Torque : robotmaniplib/Velocity Product Torque  RigidBodyTree=robot  SimulateUsing=Code generation
      settings: SourceProductBaseCode=RO
  pack joint angles : Subsystem
  tau compesation : Outport
  wires:
  pack joint angles/1(q) -> Velocity Product Torque/1, Gravity Torque/1, Inverse Dynamics/1, Forward Dynamics/1
  <jointAng>/1 -> pack joint angles/1(<jointAng>)
  pack joint angles/2(q_dot) -> Velocity Product Torque/2, Inverse Dynamics/2, Forward Dynamics/2
  Constant/1 -> Forward Dynamics/4, Inverse Dynamics/4
  Forward Dynamics/1 -> Inverse Dynamics/3
  Inverse Dynamics/1 -> tau compesation/1
  Gravity Torque/1 -> Add/1
  Velocity Product Torque/1 -> Add/2
  tau corrective/1 -> Add/3
  Add/1 -> Forward Dynamics/3

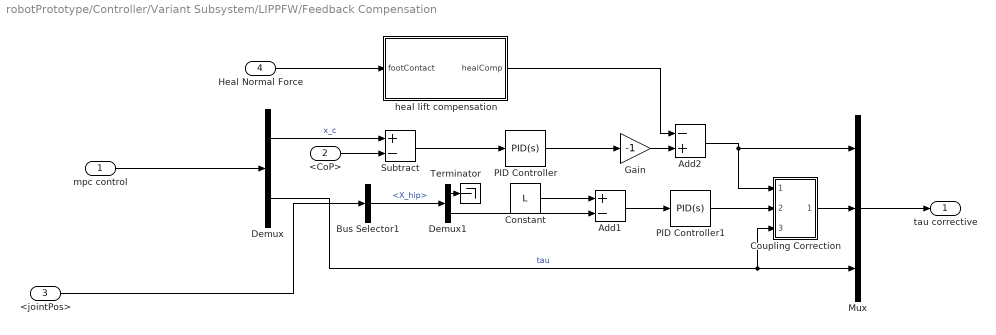
== system robotPrototype/Controller/Variant Subsystem/LIPPFW/Feedback Compensation ==
  mpc control : Inport
  <CoP> : Inport  Port=2
  <jointPos> : Inport  Port=3
  Heal Normal Force : Inport  Port=4
  Add1 : Sum  Inputs=+-
  Add2 : Sum  Inputs=-+
  Bus Selector1 : BusSelector  OutputSignals=X_hip
  Constant : Constant  Value=L
  Coupling Correction : Subsystem
  Demux : Demux  Outputs=2
  Demux1 : Demux  Outputs=2
  Gain : Gain  Gain=-1
  Mux : Mux  Inputs=3
  PID Controller : pid_lib/PID Controller  Controller=PID  Form=Parallel  TimeDomain=Continuous-time  UseExternalTs=off  SampleTime=-1  IntegratorMethod=Forward Euler  FilterMethod=Forward Euler  ControllerParametersSource=internal  P=kp_ank  I=ki_ank  D=kd_ank  UseFilter=on  N=filterCoef  TunerSelectOption=Transfer Function Based (PID Tuner App)  InitialConditionSource=internal  InitialConditionForIntegrator=0  InitialConditionForFilter=0  DifferentiatorICPrevScaledInput=0  ExternalReset=none  TrackingMode=off  Kt=1  LimitOutput=off  SatLimitsSource=internal  UpperSaturationLimit=inf  LowerSaturationLimit=-inf  LinearizeAsGain=on  AntiWindupMode=none  Kb=1  POutMin=[]  POutMax=[]  IOutMin=[]  IOutMax=[]  DOutMin=[]  DOutMax=[]  NOutMin=[]  NOutMax=[]  SumOutMin=[]  SumOutMax=[]  SaturationOutMin=[]  SaturationOutMax=[]  PParamMin=[]  PParamMax=[]  IParamMin=[]  IParamMax=[]  DParamMin=[]  DParamMax=[]  NParamMin=[]  NParamMax=[]  KbParamMin=[]  KbParamMax=[]  KtParamMin=[]  KtParamMax=[]  KbOutMin=[]  KbOutMax=[]  KtOutMin=[]  KtOutMax=[]  IntegratorOutMin=[]  IntegratorOutMax=[]  FilterOutMin=[]  FilterOutMax=[]  SumI1OutMin=[]  SumI1OutMax=[]  SumI2OutMin=[]  SumI2OutMax=[]  SumI3OutMin=[]  SumI3OutMax=[]  SumI4OutMin=[]  SumI4OutMax=[]  SumDOutMin=[]  SumDOutMax=[]  DifferentiatorOutMin=[]  DifferentiatorOutMax=[]  FilterDiffOutCoefMin=[]  FilterDiffOutCoefMax=[]  ReciprocalOutMin=[]  ReciprocalOutMax=[]  SumDenOutMin=[]  SumDenOutMax=[]  SumNumOutMin=[]  SumNumOutMax=[]  DivideOutMin=[]  DivideOutMax=[]  UdiffTsProdOutMin=[]  UdiffTsProdOutMax=[]  NTsProdOutMin=[]  NTsProdOutMax=[]  UintegralTsProdOutMin=[]  UintegralTsProdOutMax=[]  UngainTsProdOutMin=[]  UngainTsProdOutMax=[]  IntegratorContinuousStateAttributes=''  IntegratorStateMustResolveToSignalObject=off  IntegratorRTWStateStorageClass=Auto  FilterContinuousStateAttributes=''  FilterStateMustResolveToSignalObject=off  FilterRTWStateStorageClass=Auto  ParallelPVariant=InternalParameters  IdealPVariant=Disabled  IVariant=InternalParameters  DVariant=InternalParameters  IntegratorVariant=Continuous  SatVariant=Disabled  AWVariant=Passthrough  PCopyVariant=Disabled  TRVariant=Disabled  FdbkBlocksVariant=Forward  IdealPFdbkVariant=Disabled  SatFdbkVariant=Disabled  DerivativeFilterVariant=ContFilter  NVariant=InternalParameters  NCopyVariant=Disabled  FilterICVariant=InternalICsFilter  IntegratorICVariant=InternalICs  ExternalResetVariant=Disabled  TRSumVariant=Passthrough  SumFdbkVariant=Disabled  SumVariant=Sum_PID  TsampFilterVariant=InternalTs  TsampNgainVariant=Passthrough  TsampIntegralVariant=Passthrough  ExternalSaturationOutDataTypeStr=Inherit: Same as second input
  PID Controller1 : pid_lib/PID Controller  Controller=PID  Form=Parallel  TimeDomain=Continuous-time  UseExternalTs=off  SampleTime=-1  IntegratorMethod=Forward Euler  FilterMethod=Forward Euler  ControllerParametersSource=internal  P=kp_knee2  I=ki_knee2  D=kd_knee2  UseFilter=on  N=filterCoef  TunerSelectOption=Transfer Function Based (PID Tuner App)  InitialConditionSource=internal  InitialConditionForIntegrator=0  InitialConditionForFilter=0  DifferentiatorICPrevScaledInput=0  ExternalReset=none  TrackingMode=off  Kt=1  LimitOutput=off  SatLimitsSource=internal  UpperSaturationLimit=inf  LowerSaturationLimit=-inf  LinearizeAsGain=on  AntiWindupMode=none  Kb=1  POutMin=[]  POutMax=[]  IOutMin=[]  IOutMax=[]  DOutMin=[]  DOutMax=[]  NOutMin=[]  NOutMax=[]  SumOutMin=[]  SumOutMax=[]  SaturationOutMin=[]  SaturationOutMax=[]  PParamMin=[]  PParamMax=[]  IParamMin=[]  IParamMax=[]  DParamMin=[]  DParamMax=[]  NParamMin=[]  NParamMax=[]  KbParamMin=[]  KbParamMax=[]  KtParamMin=[]  KtParamMax=[]  KbOutMin=[]  KbOutMax=[]  KtOutMin=[]  KtOutMax=[]  IntegratorOutMin=[]  IntegratorOutMax=[]  FilterOutMin=[]  FilterOutMax=[]  SumI1OutMin=[]  SumI1OutMax=[]  SumI2OutMin=[]  SumI2OutMax=[]  SumI3OutMin=[]  SumI3OutMax=[]  SumI4OutMin=[]  SumI4OutMax=[]  SumDOutMin=[]  SumDOutMax=[]  DifferentiatorOutMin=[]  DifferentiatorOutMax=[]  FilterDiffOutCoefMin=[]  FilterDiffOutCoefMax=[]  ReciprocalOutMin=[]  ReciprocalOutMax=[]  SumDenOutMin=[]  SumDenOutMax=[]  SumNumOutMin=[]  SumNumOutMax=[]  DivideOutMin=[]  DivideOutMax=[]  UdiffTsProdOutMin=[]  UdiffTsProdOutMax=[]  NTsProdOutMin=[]  NTsProdOutMax=[]  UintegralTsProdOutMin=[]  UintegralTsProdOutMax=[]  UngainTsProdOutMin=[]  UngainTsProdOutMax=[]  IntegratorContinuousStateAttributes=''  IntegratorStateMustResolveToSignalObject=off  IntegratorRTWStateStorageClass=Auto  FilterContinuousStateAttributes=''  FilterStateMustResolveToSignalObject=off  FilterRTWStateStorageClass=Auto  ParallelPVariant=InternalParameters  IdealPVariant=Disabled  IVariant=InternalParameters  DVariant=InternalParameters  IntegratorVariant=Continuous  SatVariant=Disabled  AWVariant=Passthrough  PCopyVariant=Disabled  TRVariant=Disabled  FdbkBlocksVariant=Forward  IdealPFdbkVariant=Disabled  SatFdbkVariant=Disabled  DerivativeFilterVariant=ContFilter  NVariant=InternalParameters  NCopyVariant=Disabled  FilterICVariant=InternalICsFilter  IntegratorICVariant=InternalICs  ExternalResetVariant=Disabled  TRSumVariant=Passthrough  SumFdbkVariant=Disabled  SumVariant=Sum_PID  TsampFilterVariant=InternalTs  TsampNgainVariant=Passthrough  TsampIntegralVariant=Passthrough  ExternalSaturationOutDataTypeStr=Inherit: Same as second input
  Subtract : Sum  Inputs=+-
  Terminator : Terminator
  heal lift compensation : Subsystem
  tau corrective : Outport
  wires:
  Constant/1 -> Add1/1
  Demux/1 -> Subtract/1  "x_c"
  Demux/2 -> Mux/3, Coupling Correction/3(In3)  "tau"
  Subtract/1 -> PID Controller/1
  Add1/1 -> PID Controller1/1
  Demux1/1 -> Terminator/1
  Bus Selector1/1 -> Demux1/1  "<X_hip>"
  Demux1/2 -> Add1/2
  PID Controller/1 -> Gain/1
  Mux/1 -> tau corrective/1
  <jointPos>/1 -> Bus Selector1/1
  mpc control/1 -> Demux/1
  <CoP>/1 -> Subtract/2
  PID Controller1/1 -> Coupling Correction/2(In2)
  Coupling Correction/1(Output) -> Mux/2
  Gain/1 -> Add2/2
  Add2/1 -> Mux/1, Coupling Correction/1(In1)
  Heal Normal Force/1 -> heal lift compensation/1(footContact)
  heal lift compensation/1(healComp) -> Add2/1

== system robotPrototype/Controller/Variant Subsystem/LIPPFW/Inverse Dynamics ==
  tau corrective : Inport
  <jointAng> : Inport  Port=2
  Add : Sum  Inputs=+++
  Constant : Constant  Value=zeros(6,4)
  Forward Dynamics : robotmaniplib/Forward Dynamics  RigidBodyTree=robot  SimulateUsing=Code generation
  Gravity Torque : robotmaniplib/Gravity Torque  RigidBodyTree=robot  SimulateUsing=Code generation
  Inverse Dynamics : robotmaniplib/Inverse Dynamics  RigidBodyTree=robot  SimulateUsing=Code generation
      settings: SourceProductBaseCode=RO
  Velocity Product Torque : robotmaniplib/Velocity Product Torque  RigidBodyTree=robot  SimulateUsing=Code generation
      settings: SourceProductBaseCode=RO
  pack joint angles : Subsystem
  tau compesation : Outport
  wires:
  pack joint angles/1(q) -> Velocity Product Torque/1, Gravity Torque/1, Inverse Dynamics/1, Forward Dynamics/1
  pack joint angles/2(q_dot) -> Velocity Product Torque/2, Inverse Dynamics/2, Forward Dynamics/2
  Constant/1 -> Forward Dynamics/4, Inverse Dynamics/4
  Forward Dynamics/1 -> Inverse Dynamics/3
  Inverse Dynamics/1 -> tau compesation/1
  Gravity Torque/1 -> Add/1
  Velocity Product Torque/1 -> Add/2
  tau corrective/1 -> Add/3
  Add/1 -> Forward Dynamics/3
  <jointAng>/1 -> pack joint angles/1(<jointAng>)
